simulink model "PROJE_Bolum2"  (R2018b)
settings: Solver=VariableStepAuto  StartTime=0.0  StopTime=50  RelTol=1e-3
InitFcn:
  | m1=300;
  | m2=200;
  | m3=100;
  | m4=300;
  | m5=500;
  | k1=500;
  | k2=200;
  | k3=100;
  | k4=400;
  | k5=500;
  | k6=600;
  | a1=300;
  | a2=450;
  | a3=300;
  | a4=400;
  | a5=500;
  | a6=600;
  | c1=300;
  | c2=200;
  | c3=100;
  | c4=400;
  | c5=550;
  | c6=250;
  | delta1=200;
  | delta2=500;
  | delta3=400;
  | delta4=300;
  | delta5=100;
  | omega1=30;
  | omega2=50;
  | omega3=80;
  | omega4=20;
  | omega5=100;
values from neighbouring files (symbols this model uses):
  Kest1 = kalman(sysTum,Q1,R1)    [PROJE_Bolum1_Bolum2.m]
  Kest2 = kalman(sysTum,Q2,R2)    [PROJE_Bolum1_Bolum2.m]
  Kest3 = kalman(sysTum,Q3,R3)    [PROJE_Bolum1_Bolum2.m]
libraries: simulink x12
settings Model: Creator=Fatih  LastModifiedBy=Fatih

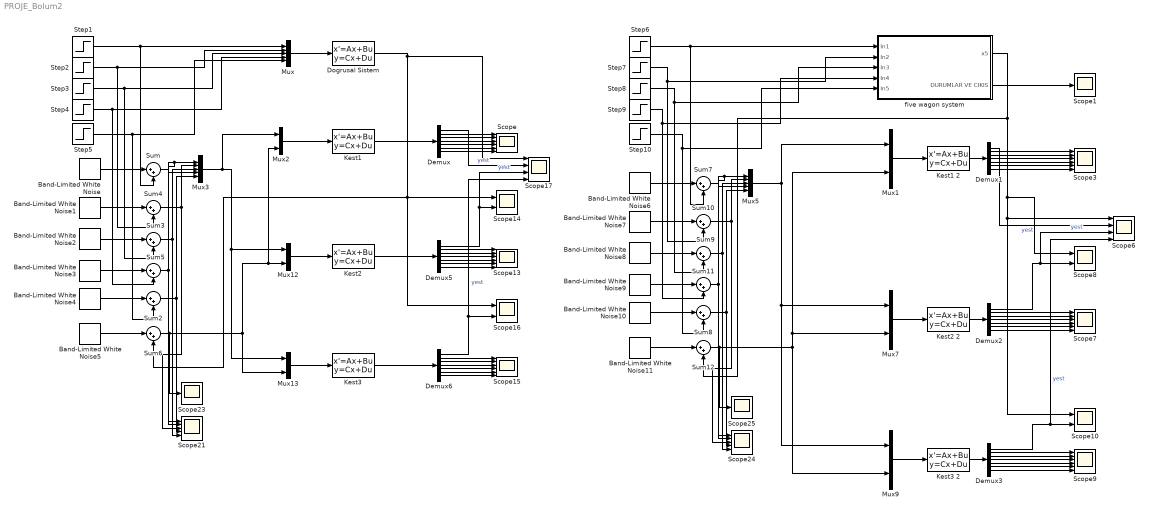
== system PROJE_Bolum2 ==
  Band-Limited White Noise{,1..5} (6 alike) : simulink/Sources/Band-Limited White Noise  Cov=[1]  Ts=0.1  seed=[23341]
  Band-Limited White Noise{6..11} (6 alike) : simulink/Sources/Band-Limited White Noise  Cov=[0.1]  Ts=0.1  seed=[23341]
  Demux{,1..3,5..6} (6 alike) : Demux  Outputs=7
  "Dogrusal Sistem " : StateSpace  A=[0 1 0 0 0 0;-2.936 -1.667 0.932 0.6667 0 0;0 0 0 1 0 0;0.5442 1 -2.359 -1.5 0 0;0 0 0 0 0 1;0 0 0.2571 4 -9.039 -5]  B=[0 0 0 0 0;0.003333 0 0 0 0;0 0 0 0 0;0 0.005 0 0 0;0 0 0 0 0;0 0 0.01 0 0]  C=[0 0 0 0 1 0]  D=[0 0 0 0 0]  InitialCondition=0
  "Kest1 " : StateSpace  A=Kest1.A  B=Kest1.B  C=Kest1.C  D=Kest1.D  InitialCondition=0
  Kest1 2 : StateSpace  A=Kest1.A  B=Kest1.B  C=Kest1.C  D=Kest1.D  InitialCondition=0
  Kest2 : StateSpace  A=Kest2.A  B=Kest2.B  C=Kest2.C  D=Kest2.D  InitialCondition=0
  Kest2 2 : StateSpace  A=Kest2.A  B=Kest2.B  C=Kest2.C  D=Kest2.D  InitialCondition=0
  Kest3 : StateSpace  A=Kest3.A  B=Kest3.B  C=Kest3.C  D=Kest3.D  InitialCondition=0
  Kest3 2 : StateSpace  A=Kest3.A  B=Kest3.B  C=Kest3.C  D=Kest3.D  InitialCondition=0
  Mux : Mux  Inputs=5
  Mux{1..2,7,9,12..13} (6 alike) : Mux  Inputs=2
  Mux3 : Mux  Inputs=5
  Mux5 : Mux  Inputs=5
  Scope{,3,7,9,13,15} (6 alike) : Scope  NumInputPorts=6
  Scope1 : Scope
  Scope{8,10,14,16} (4 alike) : Scope  NumInputPorts=2
  Scope17 : Scope  NumInputPorts=4
  Scope21 : Scope  NumInputPorts=5
  Scope23 : Scope
  Scope24 : Scope  NumInputPorts=5
  Scope25 : Scope
  Scope6 : Scope  NumInputPorts=4
  Step{1..10} (10 alike) : Step  After=100  SampleTime=0
  Sum{,2..12} (12 alike) : Sum  Inputs=|++
  "five wagon system " : Subsystem
  wires:
  Step3/1 -> Mux/3, Sum3/2
  Step1/1 -> Sum/2, Mux/1
  Step2/1 -> Mux/2, Sum4/2
  Step4/1 -> Sum5/2, Mux/4
  Step5/1 -> Sum2/2, Mux/5
  Mux3/1 -> Mux2/1, Mux13/1, Mux12/1
  "Kest1 "/1 -> Demux/1
  Mux1/1 -> Kest1 2/1
  "five wagon system "/2(DURUMLAR VE CIKIS) -> Scope1/1
  Demux/4 -> Scope/3
  Demux/3 -> Scope/2
  Demux/2 -> Scope/1
  Demux/5 -> Scope/4
  Demux/6 -> Scope/5
  Demux/7 -> Scope/6
  Kest1 2/1 -> Demux1/1
  Demux1/4 -> Scope3/3
  Demux1/7 -> Scope3/6
  Demux1/6 -> Scope3/5
  Demux1/5 -> Scope3/4
  Demux1/3 -> Scope3/2
  Demux1/2 -> Scope3/1
  Demux1/1 -> Scope6/2  "yest"
  Demux2/6 -> Scope7/5
  Demux2/7 -> Scope7/6
  Demux2/5 -> Scope7/4
  Demux2/1 -> Scope6/3, Scope8/2  "yest"
  Kest2 2/1 -> Demux2/1
  Demux2/3 -> Scope7/2
  Demux2/4 -> Scope7/3
  Demux2/2 -> Scope7/1
  Mux7/1 -> Kest2 2/1
  Kest3 2/1 -> Demux3/1
  Demux3/2 -> Scope9/1
  Demux3/1 -> Scope6/4, Scope10/2  "yest"
  Demux3/5 -> Scope9/4
  Demux3/7 -> Scope9/6
  Demux3/3 -> Scope9/2
  Demux3/6 -> Scope9/5
  Demux3/4 -> Scope9/3
  Mux9/1 -> Kest3 2/1
  Demux5/6 -> Scope13/5
  Demux5/3 -> Scope13/2
  Demux5/1 -> Scope17/3, Scope14/2  "yest"
  Kest2/1 -> Demux5/1
  Demux5/4 -> Scope13/3
  Demux5/5 -> Scope13/4
  Demux5/2 -> Scope13/1
  Demux5/7 -> Scope13/6
  Mux12/1 -> Kest2/1
  Demux6/1 -> Scope17/4, Scope16/2  "yest"
  Demux6/7 -> Scope15/6
  Demux6/2 -> Scope15/1
  Demux6/4 -> Scope15/3
  Demux6/5 -> Scope15/4
  Demux6/6 -> Scope15/5
  Demux6/3 -> Scope15/2
  Mux13/1 -> Kest3/1
  Kest3/1 -> Demux6/1
  "five wagon system "/1(x5) -> Scope10/1, Scope6/1, Scope8/1, Sum12/2
  Demux/1 -> Scope17/2  "yest"
  "Dogrusal Sistem "/1 -> Scope17/1, Sum6/2, Scope16/1, Scope14/1
  Band-Limited White Noise/1 -> Sum/1
  Sum/1 -> Mux3/1, Scope21/2
  Band-Limited White Noise1/1 -> Sum4/1
  Band-Limited White Noise2/1 -> Sum3/1
  Band-Limited White Noise3/1 -> Sum5/1
  Band-Limited White Noise4/1 -> Sum2/1
  Sum4/1 -> Mux3/2, Scope21/3
  Sum3/1 -> Mux3/3, Scope21/5
  Sum5/1 -> Mux3/4, Scope21/1
  Sum2/1 -> Mux3/5, Scope21/4
  Band-Limited White Noise5/1 -> Sum6/1
  Sum6/1 -> Mux13/2, Mux2/2, Mux12/2, Scope23/1
  Band-Limited White Noise9/1 -> Sum11/1
  Sum8/1 -> Mux5/5, Scope24/4
  Sum12/1 -> Mux9/2, Mux1/2, Mux7/2, Scope25/1
  Sum10/1 -> Mux5/2, Scope24/3
  Sum9/1 -> Mux5/3, Scope24/5
  Step6/1 -> Sum7/2, "five wagon system "/1(In1)
  Band-Limited White Noise7/1 -> Sum10/1
  Step9/1 -> Sum11/2, "five wagon system "/4(In4)
  Mux5/1 -> Mux1/1, Mux7/1, Mux9/1
  Band-Limited White Noise10/1 -> Sum8/1
  Sum11/1 -> Mux5/4, Scope24/1
  Sum7/1 -> Mux5/1, Scope24/2
  Step10/1 -> Sum8/2, "five wagon system "/5(In5)
  Band-Limited White Noise6/1 -> Sum7/1
  Step8/1 -> Sum9/2, "five wagon system "/3(In3)
  Band-Limited White Noise11/1 -> Sum12/1
  Step7/1 -> Sum10/2, "five wagon system "/2(In2)
  Band-Limited White Noise8/1 -> Sum9/1
  Mux/1 -> "Dogrusal Sistem "/1
  Mux2/1 -> "Kest1 "/1

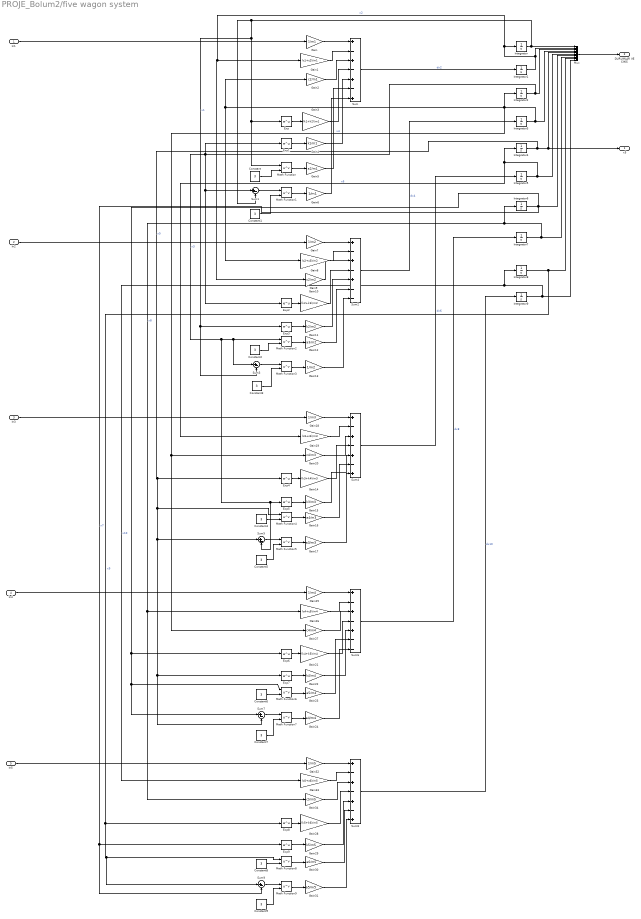
== system PROJE_Bolum2/five wagon system  ==
  In1 : Inport
  In2 : Inport  Port=2
  In3 : Inport  Port=3
  In4 : Inport  Port=4
  In5 : Inport  Port=5
  Constant{,1..9} (10 alike) : Constant  Value=3
  Exp{,1..9} (10 alike) : Math  SaturateOnIntegerOverflow=on
  Gain : Gain  Gain=1/m1
  Gain1 : Gain  Gain=(c1+c2)/m1
  Gain10 : Gain  Gain=(k2+k3)/m2
  Gain11 : Gain  Gain=k2/m2
  Gain12 : Gain  Gain=a3/m2
  Gain13 : Gain  Gain=1/m2
  Gain14 : Gain  Gain=(k3+k4)/m3
  Gain15 : Gain  Gain=k3/m3
  Gain16 : Gain  Gain=a4/m3
  Gain17 : Gain  Gain=a3/m3
  Gain18 : Gain  Gain=1/m3
  Gain19 : Gain  Gain=(c3+c4)/m3
  Gain2 : Gain  Gain=c2/m1
  Gain20 : Gain  Gain=c4/m3
  Gain21 : Gain  Gain=(k4+k5)/m4
  Gain22 : Gain  Gain=k4/m4
  Gain23 : Gain  Gain=a5/m4
  Gain24 : Gain  Gain=a4/m4
  Gain25 : Gain  Gain=1/m4
  Gain26 : Gain  Gain=(c4+c5)/m4
  Gain27 : Gain  Gain=c4/m4
  Gain28 : Gain  Gain=(k5+k6)/m5
  Gain29 : Gain  Gain=k5/m5
  Gain3 : Gain  Gain=(k1+k2)/m1
  Gain30 : Gain  Gain=a6/m5
  Gain31 : Gain  Gain=a5/m5
  Gain32 : Gain  Gain=1/m5
  Gain33 : Gain  Gain=(c5+c6)/m5
  Gain34 : Gain  Gain=c5/m5
  Gain4 : Gain  Gain=k1/m1
  Gain5 : Gain  Gain=a2/m1
  Gain6 : Gain  Gain=1/m1
  Gain7 : Gain  Gain=1/m2
  Gain8 : Gain  Gain=(c2+c3)/m2
  Gain9 : Gain  Gain=c2/m2
  Integrator{,1..9} (10 alike) : Integrator
  Math Function{,1..9} (10 alike) : Math  Operator=pow  SaturateOnIntegerOverflow=on
  Mux : Mux  Inputs=10
  Sum : Sum  Inputs=+-+-+-+
  Sum{1,3,5,7,9} (5 alike) : Sum  Inputs=|+-
  Sum2 : Sum  Inputs=+-+-+--
  Sum4 : Sum  Inputs=+-+-+-+
  Sum6 : Sum  Inputs=+-+-+--
  Sum8 : Sum  Inputs=+-+-+-+
  x5 : Outport
  DURUMLAR VE CIKIS : Outport  Port=2
  wires:
  Gain19/1 -> Sum4/2
  Constant9/1 -> Math Function9/2
  Constant8/1 -> Math Function8/2
  Exp6/1 -> Gain21/1
  Exp5/1 -> Gain15/1
  Exp9/1 -> Gain29/1
  Gain30/1 -> Sum8/6
  In2/1 -> Gain7/1
  Gain22/1 -> Sum6/5
  Math Function5/1 -> Gain17/1
  Gain20/1 -> Sum4/3
  Exp7/1 -> Gain22/1
  Gain25/1 -> Sum6/1
  Gain32/1 -> Sum8/1
  Sum5/1 -> Math Function5/1
  Constant4/1 -> Math Function4/2
  Exp4/1 -> Gain14/1
  Constant2/1 -> Math Function2/2
  Gain14/1 -> Sum4/4
  Gain16/1 -> Sum4/6
  Gain15/1 -> Sum4/5
  Gain13/1 -> Sum2/7
  Sum4/1 -> Integrator5/1  "dx6"
  Gain6/1 -> Sum/7
  Math Function1/1 -> Gain6/1
  Math Function8/1 -> Gain30/1
  Exp2/1 -> Gain10/1
  Sum9/1 -> Math Function9/1
  Gain3/1 -> Sum/4
  Sum1/1 -> Math Function1/1
  Sum8/1 -> Integrator9/1  "dx10"
  Gain24/1 -> Sum6/7
  Math Function2/1 -> Gain12/1
  In4/1 -> Gain25/1
  Constant6/1 -> Math Function6/2
  In1/1 -> Gain/1
  Gain31/1 -> Sum8/7
  Mux/1 -> DURUMLAR VE CIKIS/1
  Constant/1 -> Math Function/2
  Gain2/1 -> Sum/3
  Gain/1 -> Sum/1
  Constant7/1 -> Math Function7/2
  Math Function4/1 -> Gain16/1
  Sum3/1 -> Math Function3/1
  Sum7/1 -> Math Function7/1
  Exp1/1 -> Gain4/1
  Math Function3/1 -> Gain13/1
  Math Function6/1 -> Gain23/1
  Gain17/1 -> Sum4/7
  In5/1 -> Gain32/1
  Sum2/1 -> Integrator3/1  "dx4"
  Gain33/1 -> Sum8/2
  Integrator9/1 -> Gain33/1, Integrator8/1, Mux/10  "x10"
  Gain23/1 -> Sum6/6
  Constant5/1 -> Math Function5/2
  Gain28/1 -> Sum8/4
  In3/1 -> Gain18/1
  Integrator1/1 -> Mux/2, Gain9/1, Gain1/1, Integrator/1  "x2"
  Gain5/1 -> Sum/6
  Gain8/1 -> Sum2/2
  Gain27/1 -> Sum6/3
  Sum/1 -> Integrator1/1  "dx2"
  Sum6/1 -> Integrator7/1  "dx8"
  Gain11/1 -> Sum2/5
  Integrator7/1 -> Gain34/1, Gain26/1, Integrator6/1, Mux/8  "x8"
  Gain7/1 -> Sum2/1
  Integrator3/1 -> Integrator2/1, Gain2/1, Gain8/1, Gain27/1, Gain20/1, Mux/4  "x4"
  Gain21/1 -> Sum6/4
  Gain1/1 -> Sum/2
  Constant1/1 -> Math Function1/2
  Integrator5/1 -> Gain19/1, Integrator4/1, Mux/6  "x6"
  Gain29/1 -> Sum8/5
  Exp3/1 -> Gain11/1
  Exp/1 -> Gain3/1
  Math Function7/1 -> Gain24/1
  Gain12/1 -> Sum2/6
  Gain26/1 -> Sum6/2
  Integrator2/1 -> Mux/3, Sum5/2, Exp5/1, Sum3/1, Math Function2/1, Sum1/1, Exp2/1, Exp1/1  "x3"
  Gain9/1 -> Sum2/3
  Integrator4/1 -> Sum7/2, Exp7/1, Sum5/1, Math Function4/1, Exp4/1, x5/1, Mux/5  "x5"
  Exp8/1 -> Gain28/1
  Gain4/1 -> Sum/5
  Integrator8/1 -> Sum9/1, Math Function8/1, Exp8/1, Mux/9  "x9"
  Math Function/1 -> Gain5/1
  Gain18/1 -> Sum4/1
  Gain34/1 -> Sum8/3
  Math Function9/1 -> Gain31/1
  Integrator/1 -> Exp/1, Math Function/1, Exp3/1, Sum3/2, Sum1/2, Mux/1  "x1"
  Integrator6/1 -> Sum9/2, Exp9/1, Sum7/1, Math Function6/1, Exp6/1, Mux/7  "x7"
  Constant3/1 -> Math Function3/2
  Gain10/1 -> Sum2/4
